simulink library "lib_cosimulation"  (Simulink 4.1.1)
undefined symbols (not defined in the file or in its folder): acc_elec_eff, acc_elec_pwr, ess2_ah_nom_fun, ess2_cap_scale, ess2_dcdc_curroutmax, ess2_dcdc_eff, ess2_dcdc_vmaxout_fun, ess2_dcdc_vminin_fun, ess2_dcdc_vminout_fun, ess2_fah_max, ess2_fah_thi, ess2_fc, ess2_init_soc, ess2_max_volts, ess2_min_volts, ess2_module_num, ess2_rnom, ess2_self_disc, ess2_sg_disc, ess2_sg_full, ess2_SOC2sg, ess2_voc, ess_ah_nom_fun, ess_cap_scale, ess_fah_max, ess_fah_thi, ess_fc, ess_init_soc, ess_max_volts, ess_min_volts, ess_module_num, ess_rnom, ess_self_disc, ess_sg_disc, ess_sg_full, ess_SOC2sg, ess_voc, fc_on, gc_cutin12, gc_cutin93, gc_eff, gc_inertia, gc_map_spd, gc_max_crrnt, gc_min_volts, gc_spd_scale, gc_t12, gc_t93, gc_tempalt, gc_user_imax12, gc_user_imax93, gc_vehicletype, mc_inertia, mc_map_spd, mc_max_crrnt, mc_min_volts, mc_spd_scale, reg_temp1, reg_temp2, reg_tempreg ... (+7)
libraries: lib_cosimulation x20
(part 2 of 2)

== system lib_cosimulation/Aux Loads 14V/TurnSignals ==
  Matrix Concatenation1 : S-Function  FunctionName=smatrxcat  Parameters=numInports,catMethod  PortCounts=[]  SFunctionModules=''  mask(Matrix Concatenation){numInports=8, catMethod=Horizontal}
      mask prompts: numInports "Number of inputs:"; catMethod "Concatenation method:"
      mask help: Perform horizontal or vertical concatenation. 1-D vector input signals are treated as column vectors, i.e., [Mx1] matrices. The output is always a matrix.
      mask init:
      | xy = matrxcatmask('icon');
      mask StyleString: edit,popup(Horizontal|Vertical)
      mask Display:
      | plot(xy.x,xy.y);
      | text(0.15,0.86,xy.label);
  On6 : Constant  Value=vinf.AuxLoads.TurnSignals.On
  Product6 : Product  Inputs=2  Multiplication=Element-wise(.*)  SaturateOnIntegerOverflow=on
  Subsystem4 : lib_cosimulation/Subsystem  ModelName='TurnSignals'
  VehType : Constant  Value=vinf.AuxLoads.TurnSignals.SaberVehType
  i1 : Constant  Value=vinf.AuxLoads.TurnSignals.Data(1,2)
  i2 : Constant  Value=vinf.AuxLoads.TurnSignals.Data(2,2)
  i3 : Constant  Value=vinf.AuxLoads.TurnSignals.Data(3,2)
  v1 : Constant  Value=vinf.AuxLoads.TurnSignals.Data(1,1)
  v2 : Constant  Value=vinf.AuxLoads.TurnSignals.Data(2,1)
  v3 : Constant  Value=vinf.AuxLoads.TurnSignals.Data(3,1)
  Out1 : Outport  Port=1
  wires:
  i3/1 -> Matrix Concatenation1/7
  i2/1 -> Matrix Concatenation1/6
  i1/1 -> Matrix Concatenation1/5
  v3/1 -> Matrix Concatenation1/4
  v2/1 -> Matrix Concatenation1/3
  v1/1 -> Matrix Concatenation1/2
  Matrix Concatenation1/1 -> Out1/1
  VehType/1 -> Matrix Concatenation1/1
  Product6/1 -> Matrix Concatenation1/8
  Subsystem4/1 -> Product6/2
  On6/1 -> Product6/1

== system lib_cosimulation/Aux Loads 42V/Current Load ==
  Matrix Concatenation1 : S-Function  FunctionName=smatrxcat  Parameters=numInports,catMethod  PortCounts=[]  SFunctionModules=''  mask(Matrix Concatenation){numInports=6, catMethod=Horizontal}
      mask prompts: numInports "Number of inputs:"; catMethod "Concatenation method:"
      mask help: Perform horizontal or vertical concatenation. 1-D vector input signals are treated as column vectors, i.e., [Mx1] matrices. The output is always a matrix.
      mask init:
      | xy = matrxcatmask('icon');
      mask StyleString: edit,popup(Horizontal|Vertical)
      mask Display:
      | plot(xy.x,xy.y);
      | text(0.15,0.86,xy.label);
  i1 : Constant  Value=vinf.AuxLoads.CurrentLoad1.Data(1,2)
  i2 : Constant  Value=vinf.AuxLoads.CurrentLoad1.Data(2,2)
  i3 : Constant  Value=vinf.AuxLoads.CurrentLoad1.Data(3,2)
  v1 : Constant  Value=vinf.AuxLoads.CurrentLoad1.Data(1,1)
  v2 : Constant  Value=vinf.AuxLoads.CurrentLoad1.Data(2,1)
  v3 : Constant  Value=vinf.AuxLoads.CurrentLoad1.Data(3,1)
  Out1 : Outport  Port=1
  wires:
  Matrix Concatenation1/1 -> Out1/1
  v1/1 -> Matrix Concatenation1/1
  v2/1 -> Matrix Concatenation1/2
  v3/1 -> Matrix Concatenation1/3
  i1/1 -> Matrix Concatenation1/4
  i2/1 -> Matrix Concatenation1/5
  i3/1 -> Matrix Concatenation1/6

== system lib_cosimulation/Aux Loads 42V/Speed Load ==
  Matrix Concatenation1 : S-Function  FunctionName=smatrxcat  Parameters=numInports,catMethod  PortCounts=[]  SFunctionModules=''  mask(Matrix Concatenation){numInports=4, catMethod=Horizontal}
      mask prompts: numInports "Number of inputs:"; catMethod "Concatenation method:"
      mask help: Perform horizontal or vertical concatenation. 1-D vector input signals are treated as column vectors, i.e., [Mx1] matrices. The output is always a matrix.
      mask init:
      | xy = matrxcatmask('icon');
      mask StyleString: edit,popup(Horizontal|Vertical)
      mask Display:
      | plot(xy.x,xy.y);
      | text(0.15,0.86,xy.label);
  user_pwr1 : Constant  Value=vinf.AuxLoads.SpeedLoad1.Data(2,1)
  user_pwr2 : Constant  Value=vinf.AuxLoads.SpeedLoad1.Data(2,2)
  user_rpm1 : Constant  Value=vinf.AuxLoads.SpeedLoad1.Data(1,1)
  user_rpm2 : Constant  Value=vinf.AuxLoads.SpeedLoad1.Data(2,1)
  Out1 : Outport  Port=1
  wires:
  Matrix Concatenation1/1 -> Out1/1
  user_rpm1/1 -> Matrix Concatenation1/1
  user_rpm2/1 -> Matrix Concatenation1/2
  user_pwr1/1 -> Matrix Concatenation1/3
  user_pwr2/1 -> Matrix Concatenation1/4

== system lib_cosimulation/Aux Loads 42V/Starter ==
  Matrix Concatenation1 : lib_cosimulation/Aux Loads 14V/Starter/Matrix Concatenation1  numInports=2  catMethod=Horizontal
  Product : Product  Inputs=2  Multiplication=Element-wise(.*)  SaturateOnIntegerOverflow=on
  VehType : Constant  Value=vinf.AuxLoads.Starter.DurationOn
  VehType1 : Constant  Value=(vinf.AuxLoads.Starter.Data*vinf.AuxLoads.Starter.HiV)
  VehType3 : Constant  Value=vinf.AuxLoads.Starter.On
  Out1 : Outport  Port=1
  wires:
  VehType/1 -> Matrix Concatenation1/1
  VehType1/1 -> Product/1
  Matrix Concatenation1/1 -> Out1/1
  Product/1 -> Matrix Concatenation1/2
  VehType3/1 -> Product/2

== system lib_cosimulation/Aux Loads 42V/Starter1 ==
  14 V : Constant  Value=vinf.AuxLoads.Starter.HiV
  Hit  Crossing : HitCross  HitCrossingOffset=0  HitCrossingDirection=rising  ShowOutputPort=on
  Memory : Memory  X0=fc_on  InheritSampleTime=off
      settings: RTWStateStorageClass=Auto
  On : Constant  Value=vinf.AuxLoads.Starter.On
  On/Off : Gain  Gain=vinf.AuxLoadsOn  Multiplication=Element-wise(K.*u)  SaturateOnIntegerOverflow=on
  Product1 : Product  Inputs=4  Multiplication=Element-wise(.*)  SaturateOnIntegerOverflow=on
  Subsystem : Subsystem
      settings: RTWFcnNameOpts=Auto  RTWFileNameOpts=Auto
  Starter_OnOff_Control : Outport  Port=1
  wires:
  Memory/1 -> Hit  Crossing/1
  14 V/1 -> Product1/2
  Subsystem/1(Out1) -> Product1/3
  Product1/1 -> Starter_OnOff_Control/1
  On/1 -> On/Off/1
  [key_on] -> Product1/4
  [time] -> Subsystem/2(In2)
  [engine_on] -> Memory/1
  Hit  Crossing/1 -> Subsystem/1(In1)
  On/Off/1 -> Product1/1

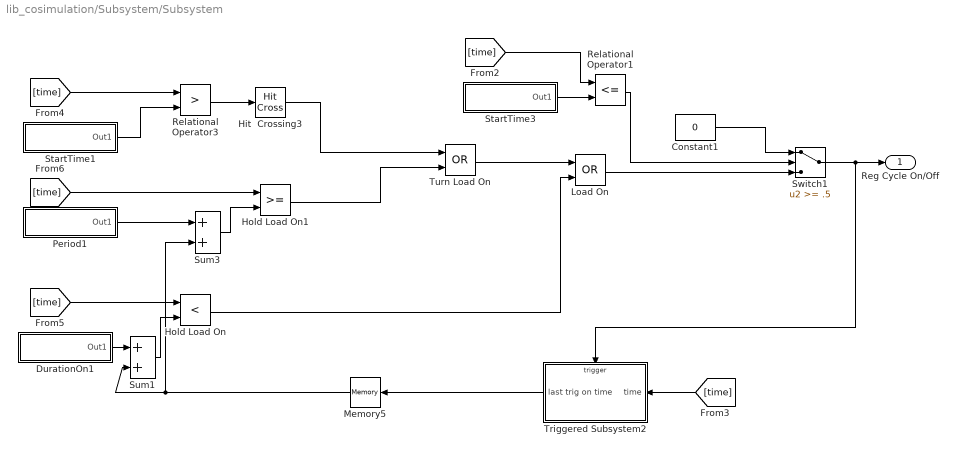
== system lib_cosimulation/Subsystem/Subsystem ==
  Constant1 : Constant  Value=0
  DurationOn1 : Subsystem  mask{ModelName=ModelName}
      mask prompts: ModelName "Auxiliary Load Model"
      mask init:
      | if (evalin('base',['isfield(vinf.AuxLoads.',ModelName,'.OnOffInfo,''DurationOn'')']) & evalin('base',['~isempty(vinf.AuxLoads.',ModelName,'.OnOffInfo.DurationOn)']));
      | DurationOn=evalin('base',['vinf.AuxLoads.',ModelName,'.OnOffInfo.DurationOn']);
      | else;DurationOn=-1;end
      settings: RTWFcnNameOpts=Auto  RTWFileNameOpts=Auto
  Hit  Crossing3 : HitCross  HitCrossingOffset=0  HitCrossingDirection=rising  ShowOutputPort=on
  Hold Load On : RelationalOperator  Operator=<
  Hold Load On1 : RelationalOperator  Operator=>=
  Load On : Logic  Operator=OR  Inputs=2
  Memory5 : Memory  Orientation=left  X0=eval('evalin(''base'',[''vinf.AuxLoads.'',ModelName,''.OnOffInfo.StartTime''])','0')  InheritSampleTime=off
      settings: RTWStateStorageClass=Auto
  Period1 : Subsystem  mask{ModelName=ModelName}
      mask prompts: ModelName "Auxiliary Load Model"
      mask init:
      | if (evalin('base',['isfield(vinf.AuxLoads.',ModelName,'.OnOffInfo,''Period'')']) & evalin('base',['~isempty(vinf.AuxLoads.',ModelName,'.OnOffInfo.Period)']));
      | Period=evalin('base',['vinf.AuxLoads.',ModelName,'.OnOffInfo.Period']);
      | else;Period=-1;end
      settings: RTWFcnNameOpts=Auto  RTWFileNameOpts=Auto
  Relational Operator1 : RelationalOperator  Operator=<=
  Relational Operator3 : RelationalOperator  Operator=>
  StartTime1 : Subsystem  mask{ModelName=ModelName}
      mask prompts: ModelName "Auxiliary Load Model"
      mask init:
      | if (evalin('base',['isfield(vinf.AuxLoads.',ModelName,'.OnOffInfo,''StartTime'')']) & evalin('base',['~isempty(vinf.AuxLoads.',ModelName,'.OnOffInfo.StartTime)']));
      | StartTime=evalin('base',['vinf.AuxLoads.',ModelName,'.OnOffInfo.StartTime']);
      | else;StartTime=-1;end
      settings: RTWFcnNameOpts=Auto  RTWFileNameOpts=Auto
  StartTime3 : Subsystem  mask{ModelName=ModelName}
      mask prompts: ModelName "Auxiliary Load Model"
      mask init: same as lib_cosimulation/Subsystem/Subsystem/StartTime1
      settings: RTWFcnNameOpts=Auto  RTWFileNameOpts=Auto
  Sum1 : Sum  Inputs=++  SaturateOnIntegerOverflow=on
  Sum3 : Sum  Inputs=++  SaturateOnIntegerOverflow=on
  Switch1 : Switch  Threshold=.5
  Triggered Subsystem2 : Subsystem  Orientation=left  TreatAsAtomicUnit=on  mask{ModelName=ModelName}
      mask prompts: ModelName "Load Name"
      mask init:
      | if (evalin('base',['isfield(vinf.AuxLoads.',ModelName,'.OnOffInfo,''StartTime'')'])); StartTime=evalin('base',['vinf.AuxLoads.',ModelName,'.OnOffInfo.StartTime']); else; StartTime=0;end
      settings: RTWFcnNameOpts=Auto  RTWFileNameOpts=Auto
  Turn Load On : Logic  Operator=OR  Inputs=2
  Reg Cycle On/Off : Outport  Port=1
  wires:
  DurationOn1/1(Out1) -> Sum1/1
  Period1/1(Out1) -> Sum3/1
  Switch1/1 -> Triggered Subsystem2/Trigger, Reg Cycle On/Off/1
  StartTime3/1(Out1) -> Relational Operator1/2
  [time] -> Relational Operator1/1
  Relational Operator1/1 -> Switch1/2
  Constant1/1 -> Switch1/1
  [time] -> Triggered Subsystem2/1(time)
  Triggered Subsystem2/1(last trig on time) -> Memory5/1
  StartTime1/1(Out1) -> Relational Operator3/2
  [time] -> Relational Operator3/1
  Relational Operator3/1 -> Hit  Crossing3/1
  [time] -> Hold Load On/1
  Sum1/1 -> Hold Load On/2
  Load On/1 -> Switch1/3
  Hold Load On1/1 -> Turn Load On/2
  Hold Load On/1 -> Load On/2
  Hit  Crossing3/1 -> Turn Load On/1
  Turn Load On/1 -> Load On/1
  [time] -> Hold Load On1/1
  Sum3/1 -> Hold Load On1/2
  Memory5/1 -> Sum3/2, Sum1/2

== system lib_cosimulation/Subsystem/Subsystem1 ==
  Memory1 : Memory  X0=0  InheritSampleTime=off
      settings: RTWStateStorageClass=Auto
  Memory3 : Memory  Orientation=left  X0=0  InheritSampleTime=off
      settings: RTWStateStorageClass=Auto
  Relational Operator1 : RelationalOperator  Operator=>
  Relational Operator2 : RelationalOperator  Operator=~=
  Sum : Sum  Inputs=+  SaturateOnIntegerOverflow=on
  ToggleTimes : Subsystem  mask{ModelName=ModelName}
      mask prompts: ModelName "Auxiliary Load Model"
      mask init:
      | if (evalin('base',['isfield(vinf.AuxLoads.',ModelName,'.OnOffInfo,''ToggleTimes'')']) & evalin('base',['~isempty(vinf.AuxLoads.',ModelName,'.OnOffInfo.ToggleTimes)']));
      | ToggleTimes=evalin('base',['vinf.AuxLoads.',ModelName,'.OnOffInfo.ToggleTimes']);
      | else;ToggleTimes=-1;end
      settings: RTWFcnNameOpts=Auto  RTWFileNameOpts=Auto
  Triggered Subsystem1 : Subsystem  TreatAsAtomicUnit=on  mask{ModelName=ModelName}
      mask prompts: ModelName "Load Name"
      mask init:
      | if (evalin('base',['isfield(vinf.AuxLoads.',ModelName,'.OnOffInfo,''InitialOn'')'])); InitialOn=evalin('base',['vinf.AuxLoads.',ModelName,'.OnOffInfo.InitialOn']);else;InitialOn=0;end
      settings: RTWFcnNameOpts=Auto  RTWFileNameOpts=Auto
  Toggle On/Off : Outport  Port=1
  wires:
  Memory1/1 -> Relational Operator2/2
  Memory3/1 -> Triggered Subsystem1/1(In1)
  Triggered Subsystem1/1(Out1) -> Toggle On/Off/1, Memory3/1
  Relational Operator2/1 -> Triggered Subsystem1/Enable
  Sum/1 -> Relational Operator2/1, Memory1/1
  Relational Operator1/1 -> Sum/1
  ToggleTimes/1(Out1) -> Relational Operator1/2
  [time] -> Relational Operator1/1

== system lib_cosimulation/14V Load Control/Starter/Subsystem ==
  In1 : Inport  Port=1  LatchInput=off
  In2 : Inport  Port=2  LatchInput=off
  Constant : Constant  Value=vinf.AuxLoads.Starter.DurationOn
  Constant1 : Constant  Value=0
  Constant2 : Constant  Value=1
  Last Engine On Time : Subsystem  TreatAsAtomicUnit=on
      settings: RTWFcnNameOpts=Auto  RTWFileNameOpts=Auto
  Relational Operator : RelationalOperator  Operator=>
  Sum : Sum  Inputs=-+  SaturateOnIntegerOverflow=on
  Switch : Switch  Threshold=.5
  Out1 : Outport  Port=1
  wires:
  Switch/1 -> Out1/1
  Constant2/1 -> Switch/1
  In1/1 -> Last Engine On Time/Trigger
  Constant1/1 -> Switch/3
  Relational Operator/1 -> Switch/2
  Last Engine On Time/1(Out1) -> Sum/1
  In2/1 -> Last Engine On Time/1(In1), Sum/2  "Current TIme"
  Sum/1 -> Relational Operator/2
  Constant/1 -> Relational Operator/1

== system lib_cosimulation/Aux Loads 14V/Starter/Starter ==
  14 V : Constant  Value=vinf.AuxLoads.Starter.V14
  Hit  Crossing : HitCross  HitCrossingOffset=0  HitCrossingDirection=rising  ShowOutputPort=on
  Memory : Memory  X0=fc_on  InheritSampleTime=off
      settings: RTWStateStorageClass=Auto
  On : Constant  Value=vinf.AuxLoads.Starter.On
  Product1 : Product  Inputs=4  Multiplication=Element-wise(.*)  SaturateOnIntegerOverflow=on
  Subsystem : Subsystem
      settings: RTWFcnNameOpts=Auto  RTWFileNameOpts=Auto
  Starter_OnOff_Control : Outport  Port=1
  wires:
  Memory/1 -> Hit  Crossing/1
  Hit  Crossing/1 -> Subsystem/1(In1)
  [engine_on] -> Memory/1
  [time] -> Subsystem/2(In2)
  [key_on] -> Product1/4
  On/1 -> Product1/1
  Product1/1 -> Starter_OnOff_Control/1
  Subsystem/1(Out1) -> Product1/3
  14 V/1 -> Product1/2

== system lib_cosimulation/Aux Loads 42V/Starter1/Subsystem ==
  In1 : Inport  Port=1  LatchInput=off
  In2 : Inport  Port=2  LatchInput=off
  Constant : Constant  Value=vinf.AuxLoads.Starter.DurationOn
  Constant1 : Constant  Value=0
  Constant2 : Constant  Value=1
  Last Engine On Time : Subsystem  TreatAsAtomicUnit=on
      settings: RTWFcnNameOpts=Auto  RTWFileNameOpts=Auto
  Relational Operator : RelationalOperator  Operator=>
  Sum : Sum  Inputs=-+  SaturateOnIntegerOverflow=on
  Switch : Switch  Threshold=.5
  Out1 : Outport  Port=1
  wires:
  Constant/1 -> Relational Operator/1
  Sum/1 -> Relational Operator/2
  In2/1 -> Sum/2, Last Engine On Time/1(In1)  "Current TIme"
  Last Engine On Time/1(Out1) -> Sum/1
  Relational Operator/1 -> Switch/2
  Constant1/1 -> Switch/3
  In1/1 -> Last Engine On Time/Trigger
  Constant2/1 -> Switch/1
  Switch/1 -> Out1/1

== system lib_cosimulation/Subsystem/Subsystem/DurationOn1 ==
  Constant : Constant  Value=DurationOn
  Out1 : Outport  Port=1
  wires:
  Constant/1 -> Out1/1

== system lib_cosimulation/Subsystem/Subsystem/Period1 ==
  Constant : Constant  Value=Period
  Out1 : Outport  Port=1
  wires:
  Constant/1 -> Out1/1

== system lib_cosimulation/Subsystem/Subsystem/StartTime1 ==
  Constant : Constant  Value=StartTime
  Out1 : Outport  Port=1
  wires:
  Constant/1 -> Out1/1

== system lib_cosimulation/Subsystem/Subsystem/StartTime3 ==
  Constant : Constant  Value=StartTime
  Out1 : Outport  Port=1
  wires:
  Constant/1 -> Out1/1

== system lib_cosimulation/Subsystem/Subsystem/Triggered Subsystem2 ==
  time : Inport  Port=1  LatchInput=off
  Trigger : TriggerPort  TriggerType=rising  OutputDataType=auto
  last trig on time : Outport  Port=1  InitialOutput=StartTime
  wires:
  time/1 -> last trig on time/1

== system lib_cosimulation/Subsystem/Subsystem1/ToggleTimes ==
  Constant : Constant  Value=ToggleTimes  VectorParams1D=off
  Out1 : Outport  Port=1
  wires:
  Constant/1 -> Out1/1

== system lib_cosimulation/Subsystem/Subsystem1/Triggered Subsystem1 ==
  In1 : Inport  Port=1  LatchInput=off
  Enable : EnablePort
  Constant1 : Constant  Value=1
  Constant2 : Constant  Value=0
  Constant3 : Constant  Value=0
  Relational Operator : RelationalOperator  Operator===
  Switch : Switch  Threshold=.5
  Out1 : Outport  Port=1  InitialOutput=InitialOn
  wires:
  In1/1 -> Relational Operator/1
  Constant2/1 -> Relational Operator/2
  Relational Operator/1 -> Switch/2
  Constant1/1 -> Switch/1
  Constant3/1 -> Switch/3
  Switch/1 -> Out1/1

== system lib_cosimulation/14V Load Control/Starter/Subsystem/Last Engine On Time ==
  In1 : Inport  Port=1  LatchInput=off
  Trigger : TriggerPort  TriggerType=rising  OutputDataType=auto
  Out1 : Outport  Port=1  InitialOutput=-100
  wires:
  In1/1 -> Out1/1

== system lib_cosimulation/Aux Loads 14V/Starter/Starter/Subsystem ==
  In1 : Inport  Port=1  LatchInput=off
  In2 : Inport  Port=2  LatchInput=off
  Constant : Constant  Value=vinf.AuxLoads.Starter.DurationOn
  Constant1 : Constant  Value=0
  Constant2 : Constant  Value=1
  Last Engine On Time : Subsystem  TreatAsAtomicUnit=on
      settings: RTWFcnNameOpts=Auto  RTWFileNameOpts=Auto
  Relational Operator : RelationalOperator  Operator=>
  Sum : Sum  Inputs=-+  SaturateOnIntegerOverflow=on
  Switch : Switch  Threshold=.5
  Out1 : Outport  Port=1
  wires:
  Switch/1 -> Out1/1
  Constant2/1 -> Switch/1
  In1/1 -> Last Engine On Time/Trigger
  Constant1/1 -> Switch/3
  Relational Operator/1 -> Switch/2
  Last Engine On Time/1(Out1) -> Sum/1
  In2/1 -> Last Engine On Time/1(In1), Sum/2  "Current TIme"
  Sum/1 -> Relational Operator/2
  Constant/1 -> Relational Operator/1

== system lib_cosimulation/Aux Loads 42V/Starter1/Subsystem/Last Engine On Time ==
  In1 : Inport  Port=1  LatchInput=off
  Trigger : TriggerPort  TriggerType=rising  OutputDataType=auto
  Out1 : Outport  Port=1  InitialOutput=-100
  wires:
  In1/1 -> Out1/1

== system lib_cosimulation/Aux Loads 14V/Starter/Starter/Subsystem/Last Engine On Time ==
  In1 : Inport  Port=1  LatchInput=off
  Trigger : TriggerPort  TriggerType=rising  OutputDataType=auto
  Out1 : Outport  Port=1  InitialOutput=-100
  wires:
  In1/1 -> Out1/1
